simulink model "course_hold_AP"  (R2017a)
settings: Solver=VariableStepAuto  StartTime=0.0  StopTime=10.0  RelTol=1e-3
values from neighbouring files (symbols this model uses):
  alpha_fi1 = 2.87    [constants.m]    (also in prob_2_e.m)
  alpha_fi2 = -0.65    [constants.m]    (also in prob_2_e.m)
  g = 9.81    [constants.m]    (also in prob_2_e.m; rlocus.m = -h)
  kd_fi = (2*zeta_fi*omega_fi-alpha_fi1)/alpha_fi2    [constants.m]    (also in prob_2_e.m)
  ki_fi = -0    (= 0)    [constants.m]    (also in prob_2_e.m)
  kp_fi = -2    [constants.m]    (also in prob_2_e.m)
  V_g = 580/3.6    (= 161.111111111)    [constants.m]    (also in prob_2_e.m)
settings Model: Creator=marti  LastModifiedBy=marti

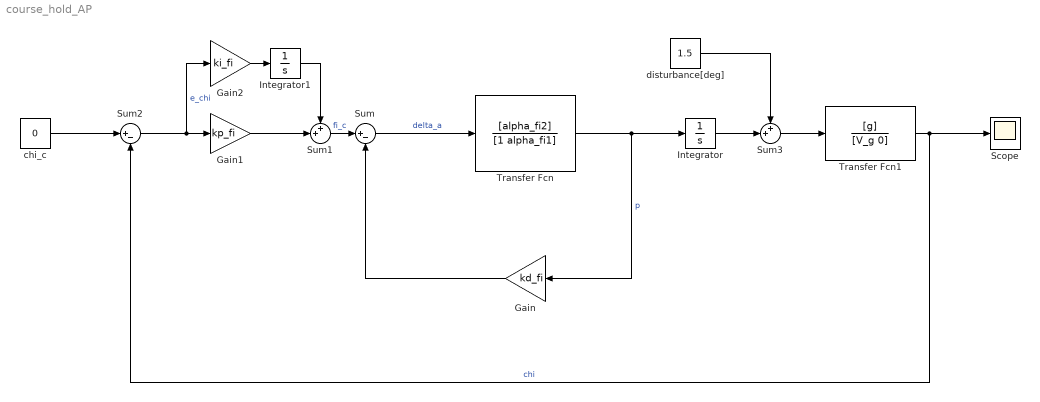
== system course_hold_AP ==
  Gain : Gain  Gain=kd_fi
  Gain1 : Gain  Gain=kp_fi
  Gain2 : Gain  Gain=ki_fi
  Integrator : Integrator
  Integrator1 : Integrator
  Scope : Scope
  Sum : Sum  Inputs=|+-
  Sum1 : Sum  Inputs=++|
  Sum2 : Sum  Inputs=|+-
  Sum3 : Sum  Inputs=++|
  Transfer Fcn : TransferFcn  Numerator=[alpha_fi2]  Denominator=[1 alpha_fi1]
  Transfer Fcn1 : TransferFcn  Numerator=[g]  Denominator=[V_g 0]
  chi_c : Constant  Value=0
  disturbance[deg] : Constant  Value=1.5
  wires:
  Transfer Fcn/1 -> Gain/1, Integrator/1  "p"
  Gain/1 -> Sum/2
  Sum/1 -> Transfer Fcn/1  "delta_a"
  Gain2/1 -> Integrator1/1
  Sum1/1 -> Sum/1  "fi_c"
  Integrator1/1 -> Sum1/1
  Gain1/1 -> Sum1/2
  Sum2/1 -> Gain2/1, Gain1/1  "e_chi"
  chi_c/1 -> Sum2/1
  Integrator/1 -> Sum3/2
  disturbance[deg]/1 -> Sum3/1
  Sum3/1 -> Transfer Fcn1/1
  Transfer Fcn1/1 -> Scope/1, Sum2/2  "chi"
